simulink model "TRAMI_DCT_AT"  (R2018b)
settings: Solver=FixedStepDiscrete  StartTime=0.0  StopTime=88  FixedStep=10e-3  RelTol=1e-3  EnableMultiTasking=on
undefined symbols (not defined in the file): CONST_AP_GEAR_SUB_NEWTRAL, CONST_AP_IDLE_SPEED_CONT, CONST_AP_LOAD_SFT, CONST_AP_LOAD_SFT_HYS, CONST_CAR_WEIGHT, CONST_CL_NUM, CONST_F_DOWN_SYNCHRO, CONST_F_SYNCHRO, CONST_F_UP_SYNCHRO, CONST_FGR, CONST_I_FlYWHEEL, CONST_INATIA_CLANK, CONST_R_SHIFT_END_CD, CONST_R_SHIFT_END_EG, CONST_R_SHIFT_END_TD, CONST_R_SHIFT_END_UP, CONST_R_SYNCHRO_ENGAGE, CONST_R_TIRE, CONST_RATIO_TQ_REDUCTION, CONST_SKIP_SHIFT_MAX, CONST_SYN_NUM, CONST_T_SFT_END_EN, CONST_T_SFT_END_JUDGE, CONST_T_SFT_END_MAX, CONST_T_SFT_END_MIN, CONST_T_SHIFT_WAIT, CONST_T_TQ_PHASE_CD, CONST_T_TQ_PHASE_ND, CONST_T_TQ_PHASE_NR, CONST_T_TQ_PHASE_TD, CONST_T_TQ_PHASE_UP, CONST_TQ_CREEP_CONT, CONST_TQ_ENGAGE_CL_MARGIN, CONST_TQ_ENGAGE_CL_MIN, CONST_TQ_INATIA_TD_SHIFT, CONST_TQ_LOAD_SFT, CONST_TQ_LOAD_SFT_HYS, CONST_TQ_ND_ENGAGE, CONST_TQ_NR_ENGAGE, CONST_TQ_TQPHASE_MIN, CONST_V_IDLE_SPEED_CONT, Eng, FALSE, GrNP, GrRev, LoopTime, MAT_CL_ENGAGE, MAT_CL_SHARE_RATE, MAT_I_ACTUATOR, MAT_SYNCHRO_COM, MAT_T_GEAR_SUB_NEWTRAL, MAT_TRANS_MGR, MaxCL, Nm, PI, Shift_CD, Shift_ND, Shift_NR, Shift_TD, Shift_Up ... (+168)
libraries: simulink x26
(part 5 of 6)

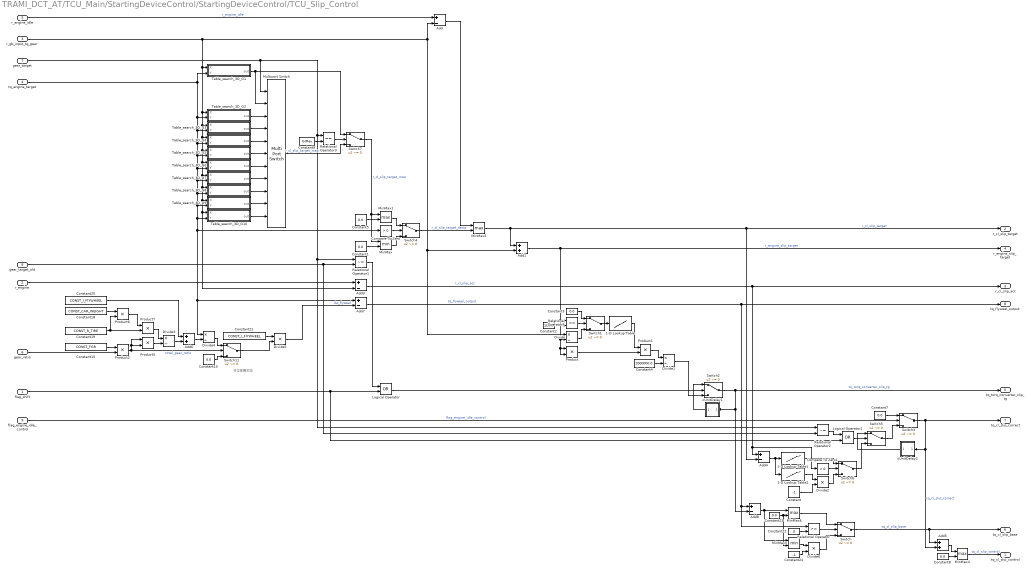
== system TRAMI_DCT_AT/TCU_Main/StartingDeviceControl/StartingDeviceControl/TCU_Slip_Control ==
  note: ゼロ除算対応
  flag_shift : Inport  OutDataTypeStr=boolean
      settings: AttributesFormatString=シフトフラグ[-]
  r_engine : Inport  Port=2  OutDataTypeStr=single
      settings: AttributesFormatString=エンジン回転数[rpm]
  r_gb_input_tg_gear : Inport  Port=3  OutDataTypeStr=single
      settings: AttributesFormatString=|
      | 目標ギヤ段でのGearBox入力回転
      | (GearBox出力回転から演算)[rpm]
  tq_engine_target : Inport  Port=4  OutDataTypeStr=single
      settings: AttributesFormatString=目標エンジントルク[Nm]
  r_engine_idle : Inport  Port=5  OutDataTypeStr=single
      settings: AttributesFormatString=エンジンアイドル回転数[rpm]
  gear_ratio : Inport  Port=6  OutDataTypeStr=single
      settings: AttributesFormatString=ギヤ比[-]
  gear_target : Inport  Port=7  OutDataTypeStr=int16
      settings: AttributesFormatString=目標ギヤ段[-]
  gear_target_old : Inport  Port=8  OutDataTypeStr=int16
      settings: AttributesFormatString=前回目標ギヤ段[-]
  flag_engine_idle_control : Inport  Port=9  OutDataTypeStr=boolean
      settings: AttributesFormatString=|
      | アイドル回転制御の実行判定フラグ
      | TRUE ：Engによるアイドル回転制御を実行
      | FALSE：クラッチスリップ制御によるEng回転制御を行う
      | [-]
  1-D Lookup Table : Lookup_n-D  NumberOfTableDimensions=1  BreakpointsForDimension1=T2D_COUPLING_CAP_FACT_X  Table=T2D_COUPLING_CAP_FACT_Y  InternalRulePriority=Speed  OutDataTypeStr=single  RndMeth=Simplest  InputSameDT=on
  1-D Lookup Table1 : Lookup_n-D  NumberOfTableDimensions=1  BreakpointsForDimension1=T2D_TQ_CL_SLIP_GAIN_X  Table=T2D_TQ_CL_SLIP_GAIN_Y  ExtrapMethod=Clip  InternalRulePriority=Speed  OutDataTypeStr=single  RndMeth=Simplest  InputSameDT=on
  1-D Lookup Table2 : Lookup_n-D  NumberOfTableDimensions=1  BreakpointsForDimension1=T2D_TQ_CL_SLIP_GAIN_X  Table=T2D_TQ_CL_SLIP_GAIN_Y  ExtrapMethod=Clip  InternalRulePriority=Speed  OutDataTypeStr=single  RndMeth=Simplest  InputSameDT=on
  Add{,3..4,8} (4 alike) : Sum  Inputs=+-  OutDataTypeStr=single
  Add1 : Sum  OutDataTypeStr=single
  Add5 : Sum  OutDataTypeStr=single
  Add6 : Sum  AccumDataTypeStr=single  OutDataTypeStr=single
  Add7 : Sum  Inputs=+-  AccumDataTypeStr=single  OutDataTypeStr=single
  Compare To Zero : simulink/Logic and Bit Operations/Compare To Zero  relop=>  OutDataTypeStr=boolean
  Compare To Zero1 : simulink/Logic and Bit Operations/Compare To Zero  relop=>  OutDataTypeStr=boolean
  Constant : Constant  Value=-1  OutDataTypeStr=single
  Constant{1,3,5,7..8,10,23} (7 alike) : Constant  Value=0.0  OutDataTypeStr=single
  Constant15 : Constant  Value=CONST_FGR  OutDataTypeStr=single
  Constant18 : Constant  Value=CONST_CAR_WEIGHT  OutDataTypeStr=single
  Constant19 : Constant  Value=CONST_R_TIRE  OutDataTypeStr=single
  Constant2 : Constant  Value=100.0  OutDataTypeStr=single
  Constant20 : Constant  Value=CONST_I_FlYWHEEL  OutDataTypeStr=single
  Constant21 : Constant  Value=CONST_I_FlYWHEEL  OutDataTypeStr=single
  Constant22 : Constant  Value=0  OutDataTypeStr=single
  Constant24 : Constant  Value=-1  OutDataTypeStr=single
  Constant4 : Constant  Value=1000000.0  OutDataTypeStr=single
  Constant9 : Constant  Value=GrRev  OutDataTypeStr=single
  Divide{,1,3..4} (4 alike) : Product  Inputs=*/  OutDataTypeStr=single
  Divide2 : Product  Inputs=**  OutDataTypeStr=single
  Divide5 : Product  Inputs=**  OutDataTypeStr=single
  Divide6 : Product  Inputs=**  OutDataTypeStr=single
  Logical Operator : Logic  Operator=OR  AllPortsSameDT=off  OutDataTypeStr=boolean
  Logical Operator1 : Logic  Operator=OR  AllPortsSameDT=off  OutDataTypeStr=boolean
  MinMax : MinMax  Inputs=2  OutDataTypeStr=single
  MinMax{1..2,4,6} (4 alike) : MinMax  Function=max  Inputs=2  OutDataTypeStr=single
  MinMax5 : MinMax  Inputs=2  OutDataTypeStr=single
  Multiport Switch : MultiPortSwitch  Inputs=9  DataPortForDefault=Additional data port  DiagnosticForDefault=None  OutDataTypeStr=single
  Product{,1..2,5..7} (6 alike) : Product  OutDataTypeStr=single
  Relational Operator : RelationalOperator  OutDataTypeStr=boolean  RndMeth=Simplest
  Relational Operator1 : RelationalOperator  Operator=~=  OutDataTypeStr=boolean  RndMeth=Nearest
  Relational Operator2 : RelationalOperator  Operator=~=  OutDataTypeStr=boolean  RndMeth=Nearest
  Relational Operator3 : RelationalOperator  Operator===  OutDataTypeStr=boolean  RndMeth=Simplest
  Relational Operator5 : RelationalOperator  Operator=<=  OutDataTypeStr=boolean  RndMeth=Nearest
  Switch{,1..7,11} (9 alike) : Switch  Criteria=u2 ~= 0  OutDataTypeStr=single
  Table_search_3D_G1 : Subsystem  mask(Table_search_3D){map=T3D_R_SLIP_G1, tbl_x=T2DX_R_SLIP_G1_Y, axis_x=T2DX_R_SLIP_G1_X, tbl_y=T2DY_R_SLIP_G1_Y, axis_y=T2DY_R_SLIP_G1_X}
      mask Display:
      | disp('Table_search_3D');
      | 
      | port_label('input',  1, 'X' );
      | port_label('input',  2, 'Y' );
      | port_label('output', 1, 'out' );
  Table_search_3D_G10 : Subsystem  mask(Table_search_3D){map=T3D_R_SLIP_G10, tbl_x=T2DX_R_SLIP_G10_Y, axis_x=T2DX_R_SLIP_G10_X, tbl_y=T2DY_R_SLIP_G10_Y, axis_y=T2DY_R_SLIP_G10_X}
      mask Display:
      | disp('Table_search_3D');
      | 
      | port_label('input',  1, 'X' );
      | port_label('input',  2, 'Y' );
      | port_label('output', 1, 'out' );
  Table_search_3D_G2 : Subsystem  mask(Table_search_3D){map=T3D_R_SLIP_G2, tbl_x=T2DX_R_SLIP_G2_Y, axis_x=T2DX_R_SLIP_G2_X, tbl_y=T2DY_R_SLIP_G2_Y, axis_y=T2DY_R_SLIP_G2_X}
      mask Display:
      | disp('Table_search_3D');
      | 
      | port_label('input',  1, 'X' );
      | port_label('input',  2, 'Y' );
      | port_label('output', 1, 'out' );
  Table_search_3D_G3 : Subsystem  mask(Table_search_3D){map=T3D_R_SLIP_G3, tbl_x=T2DX_R_SLIP_G3_Y, axis_x=T2DX_R_SLIP_G3_X, tbl_y=T2DY_R_SLIP_G3_Y, axis_y=T2DY_R_SLIP_G3_X}
      mask Display:
      | disp('Table_search_3D');
      | 
      | port_label('input',  1, 'X' );
      | port_label('input',  2, 'Y' );
      | port_label('output', 1, 'out' );
  Table_search_3D_G4 : Subsystem  mask(Table_search_3D){map=T3D_R_SLIP_G4, tbl_x=T2DX_R_SLIP_G4_Y, axis_x=T2DX_R_SLIP_G4_X, tbl_y=T2DY_R_SLIP_G4_Y, axis_y=T2DY_R_SLIP_G4_X}
      mask Display:
      | disp('Table_search_3D');
      | 
      | port_label('input',  1, 'X' );
      | port_label('input',  2, 'Y' );
      | port_label('output', 1, 'out' );
  Table_search_3D_G5 : Subsystem  mask(Table_search_3D){map=T3D_R_SLIP_G5, tbl_x=T2DX_R_SLIP_G5_Y, axis_x=T2DX_R_SLIP_G5_X, tbl_y=T2DY_R_SLIP_G5_Y, axis_y=T2DY_R_SLIP_G5_X}
      mask Display:
      | disp('Table_search_3D');
      | 
      | port_label('input',  1, 'X' );
      | port_label('input',  2, 'Y' );
      | port_label('output', 1, 'out' );
  Table_search_3D_G6 : Subsystem  mask(Table_search_3D){map=T3D_R_SLIP_G6, tbl_x=T2DX_R_SLIP_G6_Y, axis_x=T2DX_R_SLIP_G6_X, tbl_y=T2DY_R_SLIP_G6_Y, axis_y=T2DY_R_SLIP_G6_X}
      mask Display:
      | disp('Table_search_3D');
      | 
      | port_label('input',  1, 'X' );
      | port_label('input',  2, 'Y' );
      | port_label('output', 1, 'out' );
  Table_search_3D_G7 : Subsystem  mask(Table_search_3D){map=T3D_R_SLIP_G7, tbl_x=T2DX_R_SLIP_G7_Y, axis_x=T2DX_R_SLIP_G7_X, tbl_y=T2DY_R_SLIP_G7_Y, axis_y=T2DY_R_SLIP_G7_X}
      mask Display:
      | disp('Table_search_3D');
      | 
      | port_label('input',  1, 'X' );
      | port_label('input',  2, 'Y' );
      | port_label('output', 1, 'out' );
  Table_search_3D_G8 : Subsystem  mask(Table_search_3D){map=T3D_R_SLIP_G8, tbl_x=T2DX_R_SLIP_G8_Y, axis_x=T2DX_R_SLIP_G8_X, tbl_y=T2DY_R_SLIP_G8_Y, axis_y=T2DY_R_SLIP_G8_X}
      mask Display:
      | disp('Table_search_3D');
      | 
      | port_label('input',  1, 'X' );
      | port_label('input',  2, 'Y' );
      | port_label('output', 1, 'out' );
  Table_search_3D_G9 : Subsystem  mask(Table_search_3D){map=T3D_R_SLIP_G9, tbl_x=T2DX_R_SLIP_G9_Y, axis_x=T2DX_R_SLIP_G9_X, tbl_y=T2DY_R_SLIP_G9_Y, axis_y=T2DY_R_SLIP_G9_X}
      mask Display:
      | disp('Table_search_3D');
      | 
      | port_label('input',  1, 'X' );
      | port_label('input',  2, 'Y' );
      | port_label('output', 1, 'out' );
  cUnitDelay1 : Subsystem  mask(resetable_unit_delay){initParam=0}
      mask prompts: initParam "初期化値"
      mask Display: dpoly(1,[1,0],'z')
  cUnitDelay2 : Subsystem  mask(resetable_unit_delay){initParam=0}
      mask prompts: initParam "初期化値"
      mask Display: dpoly(1,[1,0],'z')
  tq_cl_slip_control : Outport  OutDataTypeStr=single
      settings: AttributesFormatString=スリップ制御クラッチのトルク容量[Nm]
  r_cl_slip_target : Outport  Port=2  OutDataTypeStr=single
      settings: AttributesFormatString=目標スリップ量[rpm]
  r_cl_slip_act : Outport  Port=3  OutDataTypeStr=single
      settings: AttributesFormatString=実スリップ量[rpm]
  r_engine_slip_target : Outport  Port=4  OutDataTypeStr=single
      settings: AttributesFormatString=目標エンジン回転[rpm]
  tq_torq_converter_slip_tg : Outport  Port=5  OutDataTypeStr=single
      settings: AttributesFormatString=目標スリップ時の流体伝達トルク[Nm]
  tq_cl_slip_base : Outport  Port=6  OutDataTypeStr=single
      settings: AttributesFormatString=スリップクラッチのトルク容量基準値[Nm]
  tq_cl_slip_correct : Outport  Port=7  OutDataTypeStr=single
      settings: AttributesFormatString=クラッチトルクの補正値[Nm]
  tq_flyweel_output : Outport  Port=8  OutDataTypeStr=single
      settings: AttributesFormatString=イナーシャを考慮したフライホイール出力トルク[Nm]
  wires:
  r_gb_input_tg_gear/1 -> Add3/2, Table_search_3D_G10/1(X), Table_search_3D_G9/1(X), Table_search_3D_G8/1(X), Table_search_3D_G7/1(X), Table_search_3D_G6/1(X), Table_search_3D_G5/1(X), Table_search_3D_G4/1(X), Table_search_3D_G3/1(X), Table_search_3D_G2/1(X), Table_search_3D_G1/1(X), Add1/2, Divide/1, Add/2
  gear_target/1 -> Multiport Switch/1, Relational Operator1/1, Relational Operator2/1, Relational Operator3/1
  Table_search_3D_G1/1(out) -> Multiport Switch/2, Switch7/1
  Table_search_3D_G2/1(out) -> Multiport Switch/3
  Table_search_3D_G3/1(out) -> Multiport Switch/4
  Table_search_3D_G4/1(out) -> Multiport Switch/5
  Table_search_3D_G5/1(out) -> Multiport Switch/6
  Table_search_3D_G6/1(out) -> Multiport Switch/7
  Table_search_3D_G7/1(out) -> Multiport Switch/8
  Table_search_3D_G8/1(out) -> Multiport Switch/9
  Table_search_3D_G9/1(out) -> Multiport Switch/10
  Table_search_3D_G10/1(out) -> Multiport Switch/11
  tq_engine_target/1 -> Compare To Zero/1, Divide4/1, Add7/1, Table_search_3D_G10/2(Y), Table_search_3D_G9/2(Y), Table_search_3D_G8/2(Y), Table_search_3D_G7/2(Y), Table_search_3D_G6/2(Y), Table_search_3D_G5/2(Y), Table_search_3D_G4/2(Y), Table_search_3D_G3/2(Y), Table_search_3D_G2/2(Y), Table_search_3D_G1/2(Y)
  Switch7/1 -> MinMax/1, MinMax1/1  "r_cl_slip_target_map"
  Compare To Zero/1 -> Switch4/2
  MinMax1/1 -> Switch4/1
  MinMax/1 -> Switch4/3
  Constant5/1 -> MinMax1/2
  Constant1/1 -> MinMax/2
  Switch4/1 -> MinMax2/2  "r_cl_slip_target_temp"
  Add/1 -> MinMax2/1
  r_engine_idle/1 -> Add/1  "r_engine_idle"
  Add1/1 -> r_engine_slip_target/1, Relational Operator5/1, Product/2, Product/1, Divide/2  "r_engine_slip_target"
  Constant2/1 -> Relational Operator5/2
  Relational Operator5/1 -> Switch1/2
  Constant3/1 -> Switch1/1
  Switch1/1 -> 1-D Lookup Table/1
  Divide/1 -> Switch1/3
  1-D Lookup Table/1 -> Product1/1
  Relational Operator1/1 -> Logical Operator/1
  flag_shift/1 -> Logical Operator/2, Logical Operator1/2
  Logical Operator/1 -> Switch2/2
  Switch2/1 -> cUnitDelay1/1(<param>), Add8/2, tq_torq_converter_slip_tg/1  "tq_torq_converter_slip_tg"
  Product1/1 -> Divide1/1
  Constant4/1 -> Divide1/2
  Product/1 -> Product1/2
  Divide1/1 -> Switch2/3
  r_engine/1 -> Add3/1
  Switch3/1 -> tq_cl_slip_correct/1, Add5/2, cUnitDelay2/1(<param>)  "tq_cl_slip_correct"
  Switch5/1 -> Switch3/3
  Switch6/1 -> Switch5/3
  flag_engine_idle_control/1 -> Switch3/2  "flag_engine_idle_control"
  Constant7/1 -> Switch3/1
  cUnitDelay2/1(preParam) -> Switch5/1
  Logical Operator1/1 -> Switch5/2
  Relational Operator2/1 -> Logical Operator1/1
  Compare To Zero1/1 -> Switch6/2
  Add3/1 -> r_cl_slip_act/1, Compare To Zero1/1, Add4/1  "r_cl_slip_act"
  1-D Lookup Table2/1 -> Divide2/1
  Add4/1 -> 1-D Lookup Table1/1, 1-D Lookup Table2/1
  MinMax2/1 -> r_cl_slip_target/1, Add4/2, Add1/1  "r_cl_slip_target"
  MinMax4/1 -> tq_cl_slip_control/1  "tq_cl_slip_control"
  Add5/1 -> MinMax4/1
  Constant8/1 -> MinMax4/2
  gear_target_old/1 -> Relational Operator2/2, Relational Operator1/2
  Constant/1 -> Divide2/2
  Divide2/1 -> Switch6/3
  1-D Lookup Table1/1 -> Switch6/1
  Constant15/1 -> Product2/1
  gear_ratio/1 -> Product2/2
  Add6/1 -> Divide4/2
  Product2/1 -> Product5/1, Product5/2, Switch11/2  "total_gear_ratio"
  Constant18/1 -> Product6/1
  Constant19/1 -> Product6/2, Product7/2
  Product6/1 -> Product7/1
  Product7/1 -> Divide3/1
  Constant20/1 -> Add6/1
  Switch11/1 -> Divide5/2
  Constant21/1 -> Divide5/1
  Divide5/1 -> Add7/2  "dw_flyweel"
  Add7/1 -> tq_flyweel_output/1, Add8/1, Relational Operator/1  "tq_flyweel_output"
  Relational Operator/1 -> Switch/2
  Constant22/1 -> Relational Operator/2
  MinMax6/1 -> Switch/1
  Divide6/1 -> Switch/3
  Add8/1 -> MinMax6/1, MinMax5/1
  Constant23/1 -> MinMax5/2, MinMax6/2
  Constant24/1 -> Divide6/2
  MinMax5/1 -> Divide6/1
  Switch/1 -> tq_cl_slip_base/1, Add5/1  "tq_cl_slip_base"
  Divide3/1 -> Add6/2
  Product5/1 -> Divide3/2
  Divide4/1 -> Switch11/1
  cUnitDelay1/1(preParam) -> Switch2/1
  Relational Operator3/1 -> Switch7/2
  Constant9/1 -> Relational Operator3/2
  Multiport Switch/1 -> Switch7/3  "r_cl_slip_target_map"
  Constant10/1 -> Switch11/3

== system TRAMI_DCT_AT/TCU_Main/StartingDeviceControl/StartingDeviceControl/TCU_Torque_Input_GearBox ==
  tq_engine_target : Inport  OutDataTypeStr=single
      settings: AttributesFormatString=目標エンジントルク[Nm]
  torq_ratio_torq_converter : Inport  Port=2  OutDataTypeStr=single
      settings: AttributesFormatString=トルク比[-]
  Divide : Product  Inputs=**  OutDataTypeStr=single
  tq_gearbox_input : Outport  OutDataTypeStr=single
      settings: AttributesFormatString=ギヤボックス入力トルク[Nm]
  wires:
  tq_engine_target/1 -> Divide/1
  torq_ratio_torq_converter/1 -> Divide/2
  Divide/1 -> tq_gearbox_input/1  "tq_gearbox_input"

== system TRAMI_DCT_AT/TCU_Main/AccControl/AccControl/TCU_EOP_Control/Table_search_3D_sample6 ==
  X : Inport  OutDataTypeStr=single
  Y : Inport  Port=2  OutDataTypeStr=single
  1-D Lookup Table1 : Lookup_n-D  NumberOfTableDimensions=1  BreakpointsForDimension1=axis_x  Table=tbl_x  ExtrapMethod=Clip  InternalRulePriority=Speed  OutDataTypeStr=single  RndMeth=Simplest  InputSameDT=on
  1-D Lookup Table2 : Lookup_n-D  NumberOfTableDimensions=1  BreakpointsForDimension1=axis_y  Table=tbl_y  ExtrapMethod=Clip  InternalRulePriority=Speed  OutDataTypeStr=single  RndMeth=Simplest  InputSameDT=on
  2-D Lookup Table : Lookup_n-D  BreakpointsForDimension1=tbl_y  BreakpointsForDimension2=tbl_x  Table=map  ExtrapMethod=Clip  InternalRulePriority=Speed  OutDataTypeStr=single  RndMeth=Simplest  InputSameDT=on
  out : Outport  OutDataTypeStr=single
  wires:
  1-D Lookup Table1/1 -> 2-D Lookup Table/2  "x_nrm"
  1-D Lookup Table2/1 -> 2-D Lookup Table/1  "y_nrm"
  Y/1 -> 1-D Lookup Table2/1  "data_y"
  X/1 -> 1-D Lookup Table1/1  "data_x"
  2-D Lookup Table/1 -> out/1

== system TRAMI_DCT_AT/TCU_Main/ClutchControl/ClutchControl/TCU_Gear_Clutch_Control/cUnitDelay2 ==
  <param> : Inport
  Constant13 : Constant  Value=initParam  OutDataTypeStr=int16
  Switch12 : Switch  Criteria=u2 > Threshold
  Unit Delay2 : UnitDelay  InitialCondition=zeros(size(initParam))  SampleTime=-1
  preParam : Outport
  wires:
  Unit Delay2/1 -> Switch12/3
  Switch12/1 -> preParam/1
  [FlagInit] -> Switch12/2
  Constant13/1 -> Switch12/1
  <param>/1 -> Unit Delay2/1

== system TRAMI_DCT_AT/TCU_Main/ClutchControl/ClutchControl/TCU_SYNCHORO_CONTROL_AT_DCT/TCU_SYNCHORO_CONTROL_AT ==
  gear_target : Inport  OutDataTypeStr=int16
      settings: AttributesFormatString=目標ギヤ段[-]
  gear_before_shift : Inport  Port=2  OutDataTypeStr=int16
      settings: AttributesFormatString=変速前ギヤ段[-]
  gear_sub1 : Inport  Port=3  OutDataTypeStr=int16
      settings: AttributesFormatString=待機ギヤ段（奇数軸）[-]
  gear_sub2 : Inport  Port=4  OutDataTypeStr=int16
      settings: AttributesFormatString=待機ギヤ段（偶数軸）[-]
  f_synchro_old : Inport  Port=5  OutDataTypeStr=single
      settings: AttributesFormatString=前回のシンクロの押し力[N]
  Constant1 : Constant  Value=[0 0 0 0 0 0 0 0 0 0]  OutDataTypeStr=single
  Constant13 : Constant  Value=FALSE  OutDataTypeStr=boolean
  Terminator{,1..4} (5 alike) : Terminator
  f_synchro : Outport  OutDataTypeStr=single
      settings: AttributesFormatString=シンクロの押し力[N]
  flag_synchro_com : Outport  Port=2  OutDataTypeStr=boolean
      settings: AttributesFormatString=シンクロ締結指示[-]
  wires:
  gear_before_shift/1 -> Terminator1/1
  gear_target/1 -> Terminator/1
  Constant13/1 -> flag_synchro_com/1  "flag_synchro_com"
  Constant1/1 -> f_synchro/1  "f_synchro"
  gear_sub1/1 -> Terminator2/1
  gear_sub2/1 -> Terminator3/1
  f_synchro_old/1 -> Terminator4/1

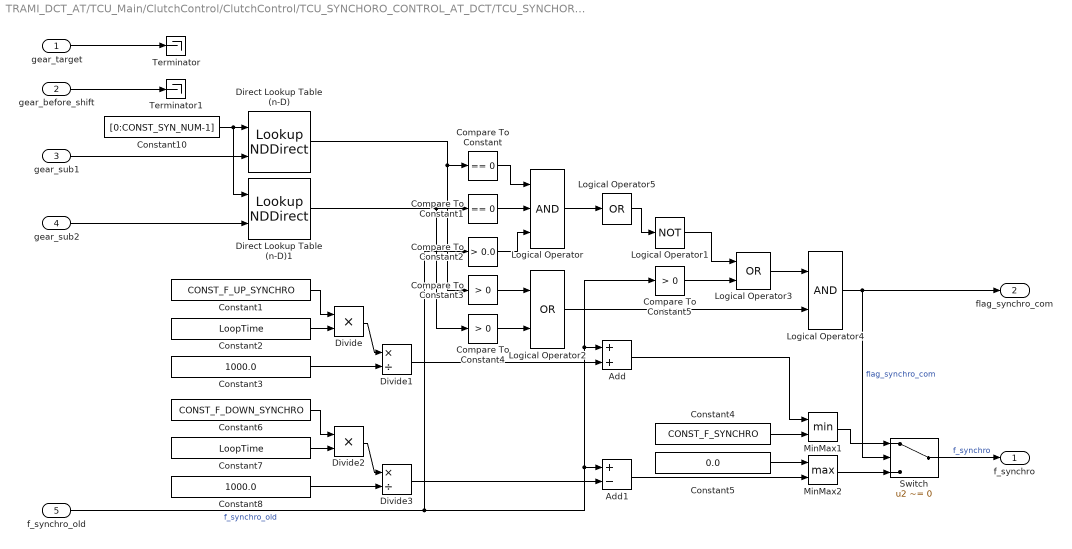
== system TRAMI_DCT_AT/TCU_Main/ClutchControl/ClutchControl/TCU_SYNCHORO_CONTROL_AT_DCT/TCU_SYNCHORO_CONTROL_DCT ==
  gear_target : Inport  OutDataTypeStr=int16
      settings: AttributesFormatString=目標ギヤ段[-]
  gear_before_shift : Inport  Port=2  OutDataTypeStr=int16
      settings: AttributesFormatString=変速前ギヤ段[-]
  gear_sub1 : Inport  Port=3  OutDataTypeStr=int16
      settings: AttributesFormatString=待機ギヤ段（奇数軸）[-]
  gear_sub2 : Inport  Port=4  OutDataTypeStr=int16
      settings: AttributesFormatString=待機ギヤ段（偶数軸）[-]
  f_synchro_old : Inport  Port=5  OutDataTypeStr=single
      settings: AttributesFormatString=前回のシンクロの押し力[N]
  Add : Sum  OutDataTypeStr=single
  Add1 : Sum  Inputs=+-  OutDataTypeStr=single
  Compare To Constant : simulink/Logic and Bit Operations/Compare To Constant  relop===  const=0  OutDataTypeStr=boolean
  Compare To Constant1 : simulink/Logic and Bit Operations/Compare To Constant  relop===  const=0  OutDataTypeStr=boolean
  Compare To Constant2 : simulink/Logic and Bit Operations/Compare To Constant  relop=>  const=0.0  OutDataTypeStr=boolean
  Compare To Constant3 : simulink/Logic and Bit Operations/Compare To Constant  relop=>  const=0  OutDataTypeStr=boolean
  Compare To Constant4 : simulink/Logic and Bit Operations/Compare To Constant  relop=>  const=0  OutDataTypeStr=boolean
  Compare To Constant5 : simulink/Logic and Bit Operations/Compare To Constant  relop=>  const=0  OutDataTypeStr=boolean
  Constant1 : Constant  Value=CONST_F_UP_SYNCHRO  OutDataTypeStr=single
  Constant10 : Constant  Value=[0:CONST_SYN_NUM-1]  OutDataTypeStr=int16
  Constant2 : Constant  Value=LoopTime  OutDataTypeStr=single
  Constant3 : Constant  Value=1000.0  OutDataTypeStr=single
  Constant4 : Constant  Value=CONST_F_SYNCHRO  OutDataTypeStr=single
  Constant5 : Constant  Value=0.0  OutDataTypeStr=single
  Constant6 : Constant  Value=CONST_F_DOWN_SYNCHRO  OutDataTypeStr=single
  Constant7 : Constant  Value=LoopTime  OutDataTypeStr=single
  Constant8 : Constant  Value=1000.0  OutDataTypeStr=single
  Direct Lookup Table (n-D) : LookupNDDirect  Table=MAT_SYNCHRO_COM
  Direct Lookup Table (n-D)1 : LookupNDDirect  Table=MAT_SYNCHRO_COM
  Divide : Product  OutDataTypeStr=single
  Divide1 : Product  Inputs=*/  OutDataTypeStr=single
  Divide2 : Product  OutDataTypeStr=single
  Divide3 : Product  Inputs=*/  OutDataTypeStr=single
  Logical Operator : Logic  Inputs=3  AllPortsSameDT=off  OutDataTypeStr=boolean
  Logical Operator1 : Logic  Operator=NOT  Inputs=3  AllPortsSameDT=off  OutDataTypeStr=boolean
  Logical Operator2 : Logic  Operator=OR  AllPortsSameDT=off  OutDataTypeStr=boolean
  Logical Operator3 : Logic  Operator=OR  AllPortsSameDT=off  OutDataTypeStr=boolean
  Logical Operator4 : Logic  AllPortsSameDT=off  OutDataTypeStr=boolean
  Logical Operator5 : Logic  Operator=OR  Inputs=1  AllPortsSameDT=off  OutDataTypeStr=boolean
  MinMax1 : MinMax  Inputs=2  OutDataTypeStr=single
  MinMax2 : MinMax  Function=max  Inputs=2  OutDataTypeStr=single
  Switch : Switch  Criteria=u2 ~= 0  OutDataTypeStr=single  ZeroCross=off
  Terminator : Terminator
  Terminator1 : Terminator
  f_synchro : Outport  OutDataTypeStr=single
      settings: AttributesFormatString=シンクロの押し力[N]
  flag_synchro_com : Outport  Port=2  OutDataTypeStr=boolean
      settings: AttributesFormatString=シンクロ締結指示[-]
  wires:
  Constant5/1 -> MinMax2/1
  Logical Operator4/1 -> Switch/2, flag_synchro_com/1  "flag_synchro_com"
  Constant3/1 -> Divide1/2
  Compare To Constant4/1 -> Logical Operator2/2
  Constant8/1 -> Divide3/2
  Logical Operator1/1 -> Logical Operator3/1
  Logical Operator5/1 -> Logical Operator1/1
  gear_target/1 -> Terminator/1
  Compare To Constant2/1 -> Logical Operator/3
  gear_before_shift/1 -> Terminator1/1
  Compare To Constant1/1 -> Logical Operator/2
  Compare To Constant3/1 -> Logical Operator2/1
  Switch/1 -> f_synchro/1  "f_synchro"
  Direct Lookup Table (n-D)/1 -> Compare To Constant3/1, Compare To Constant/1
  Logical Operator2/1 -> Logical Operator4/2
  Constant1/1 -> Divide/1
  Divide2/1 -> Divide3/1
  Constant10/1 -> Direct Lookup Table (n-D)/1, Direct Lookup Table (n-D)1/1
  Constant6/1 -> Divide2/1
  gear_sub2/1 -> Direct Lookup Table (n-D)1/2
  gear_sub1/1 -> Direct Lookup Table (n-D)/2
  Constant7/1 -> Divide2/2
  Add/1 -> MinMax1/1
  Compare To Constant/1 -> Logical Operator/1
  Add1/1 -> MinMax2/2
  Logical Operator3/1 -> Logical Operator4/1
  Compare To Constant5/1 -> Logical Operator3/2
  Divide3/1 -> Add1/2
  Direct Lookup Table (n-D)1/1 -> Compare To Constant4/1, Compare To Constant1/1
  Divide1/1 -> Add/2
  Constant4/1 -> MinMax1/2
  MinMax2/1 -> Switch/3
  MinMax1/1 -> Switch/1
  Logical Operator/1 -> Logical Operator5/1
  Divide/1 -> Divide1/1
  f_synchro_old/1 -> Compare To Constant5/1, Add/1, Add1/1, Compare To Constant2/1  "f_synchro_old"
  Constant2/1 -> Divide/2

== system TRAMI_DCT_AT/TCU_Main/ClutchControl/ClutchControl/TCU_SYNCHORO_STATUS_AT_DCT/TCU_SYNCHORO_STATUS_AT ==
  gear_target : Inport  OutDataTypeStr=int16
      settings: AttributesFormatString=目標ギヤ段[-]
  f_synchro : Inport  Port=2  OutDataTypeStr=single
      settings: AttributesFormatString=シンクロの押し力[N]
  r_synchoro_dif : Inport  Port=3  OutDataTypeStr=single
      settings: AttributesFormatString=各シンクロ差回転[rpm]
  Constant : Constant  Value=TRUE  OutDataTypeStr=boolean
  Terminator : Terminator
  Terminator1 : Terminator
  Terminator2 : Terminator
  flag_synchro_ready : Outport  OutDataTypeStr=boolean
      settings: AttributesFormatString=全シンクロの同期判定[-]
  wires:
  Constant/1 -> flag_synchro_ready/1  "flag_synchro_ready"
  gear_target/1 -> Terminator/1  "gear_target"
  f_synchro/1 -> Terminator1/1  "f_synchro"
  r_synchoro_dif/1 -> Terminator2/1  "r_synchoro_dif"

== system TRAMI_DCT_AT/TCU_Main/ClutchControl/ClutchControl/TCU_SYNCHORO_STATUS_AT_DCT/TCU_SYNCHORO_STATUS_DCT ==
  gear_target : Inport  OutDataTypeStr=int16
      settings: AttributesFormatString=目標ギヤ段[-]
  f_synchro : Inport  Port=2  OutDataTypeStr=single
      settings: AttributesFormatString=シンクロの押し力[N]
  r_synchoro_dif : Inport  Port=3  OutDataTypeStr=single
      settings: AttributesFormatString=各シンクロ差回転[rpm]
  Abs : Abs  OutDataTypeStr=single
  Compare To Constant : simulink/Logic and Bit Operations/Compare To Constant  relop=>  const=0  OutDataTypeStr=boolean
  Constant10 : Constant  Value=CONST_R_SYNCHRO_ENGAGE  OutDataTypeStr=single
  Constant3 : Constant  Value=[0:CONST_SYN_NUM-1]  OutDataTypeStr=int16
  Constant9 : Constant  Value=CONST_F_SYNCHRO  OutDataTypeStr=single
  Direct Lookup Table (n-D) : LookupNDDirect  Table=MAT_SYNCHRO_COM
  Logical Operator : Logic  AllPortsSameDT=off  OutDataTypeStr=boolean
  Logical Operator1 : Logic  Operator=NOT  Inputs=3  AllPortsSameDT=off  OutDataTypeStr=boolean
  Logical Operator5 : Logic  Operator=OR  Inputs=1  AllPortsSameDT=off  OutDataTypeStr=boolean
  Logical Operator6 : Logic  Operator=OR  AllPortsSameDT=off  OutDataTypeStr=boolean
  Relational Operator : RelationalOperator  Operator=<  OutDataTypeStr=boolean  RndMeth=Nearest
  Relational Operator1 : RelationalOperator  Operator=>  OutDataTypeStr=boolean  RndMeth=Nearest
  Selector1 : Selector  InputPortWidth=MaxSyn  IndexOptions=Index vector (dialog)  Indices=[1:CONST_SYN_NUM]  OutputSizes=1
  flag_synchro_ready : Outport  OutDataTypeStr=boolean
      settings: AttributesFormatString=全シンクロの同期判定[-]
  wires:
  r_synchoro_dif/1 -> Selector1/1  "r_synchoro_dif"
  Logical Operator/1 -> Logical Operator5/1
  Logical Operator5/1 -> Logical Operator1/1
  Logical Operator6/1 -> Logical Operator/2
  Logical Operator1/1 -> flag_synchro_ready/1  "flag_synchro_ready"
  Constant3/1 -> Direct Lookup Table (n-D)/1
  gear_target/1 -> Direct Lookup Table (n-D)/2  "gear_target"
  Relational Operator1/1 -> Logical Operator6/2
  Constant10/1 -> Relational Operator1/2
  f_synchro/1 -> Relational Operator/1  "f_synchro"
  Relational Operator/1 -> Logical Operator6/1
  Compare To Constant/1 -> Logical Operator/1
  Abs/1 -> Relational Operator1/1
  Constant9/1 -> Relational Operator/2
  Direct Lookup Table (n-D)/1 -> Compare To Constant/1
  Selector1/1 -> Abs/1

== system TRAMI_DCT_AT/TCU_Main/ClutchControl/ClutchControl/TCU_Shift_Inertia_Torq/cUnitDelay1 ==
  <param> : Inport
  Constant13 : Constant  Value=initParam  OutDataTypeStr=single
  Switch12 : Switch  Criteria=u2 > Threshold
  Unit Delay2 : UnitDelay  InitialCondition=zeros(size(initParam))  SampleTime=-1
  preParam : Outport
  wires:
  Unit Delay2/1 -> Switch12/3
  Switch12/1 -> preParam/1
  [FlagInit] -> Switch12/2
  Constant13/1 -> Switch12/1
  <param>/1 -> Unit Delay2/1

== system TRAMI_DCT_AT/TCU_Main/ClutchControl/ClutchControl/TCU_Shift_Inertia_Torq/cUnitDelay2 ==
  <param> : Inport
  Constant13 : Constant  Value=initParam  OutDataTypeStr=single
  Switch12 : Switch  Criteria=u2 > Threshold
  Unit Delay2 : UnitDelay  InitialCondition=zeros(size(initParam))  SampleTime=-1
  preParam : Outport
  wires:
  Unit Delay2/1 -> Switch12/3
  Switch12/1 -> preParam/1
  [FlagInit] -> Switch12/2
  Constant13/1 -> Switch12/1
  <param>/1 -> Unit Delay2/1

== system TRAMI_DCT_AT/TCU_Main/ClutchControl/ClutchControl/TCU_Shift_Inertia_Torq/cUnitDelay3 ==
  <param> : Inport
  Constant13 : Constant  Value=initParam  OutDataTypeStr=int16
  Switch12 : Switch  Criteria=u2 > Threshold
  Unit Delay2 : UnitDelay  InitialCondition=zeros(size(initParam))  SampleTime=-1
  preParam : Outport
  wires:
  <param>/1 -> Unit Delay2/1
  Constant13/1 -> Switch12/1
  [FlagInit] -> Switch12/2
  Switch12/1 -> preParam/1
  Unit Delay2/1 -> Switch12/3

== system TRAMI_DCT_AT/TCU_Main/ClutchControl/ClutchControl/TCU_Shift_Inertia_Torq/cUnitDelay4 ==
  <param> : Inport
  Constant13 : Constant  Value=initParam  OutDataTypeStr=single
  Switch12 : Switch  Criteria=u2 > Threshold
  Unit Delay2 : UnitDelay  InitialCondition=zeros(size(initParam))  SampleTime=-1
  preParam : Outport
  wires:
  <param>/1 -> Unit Delay2/1
  Constant13/1 -> Switch12/1
  [FlagInit] -> Switch12/2
  Switch12/1 -> preParam/1
  Unit Delay2/1 -> Switch12/3

== system TRAMI_DCT_AT/TCU_Main/GearControl/GearControl/TCU_Up_Shift_Torque_Reduction/cUnitDelay2 ==
  <param> : Inport
  Constant13 : Constant  Value=initParam  OutDataTypeStr=boolean
  Switch12 : Switch  Criteria=u2 > Threshold
  Unit Delay2 : UnitDelay  InitialCondition=zeros(size(initParam))  SampleTime=-1
  preParam : Outport
  wires:
  Unit Delay2/1 -> Switch12/3
  Switch12/1 -> preParam/1
  [FlagInit] -> Switch12/2
  Constant13/1 -> Switch12/1
  <param>/1 -> Unit Delay2/1

== system TRAMI_DCT_AT/TCU_Main/ShiftScheduleControl/ShiftScheduleControl/TCU_Gear_Shift_Type/cUnitDelay2 ==
  <param> : Inport
  Constant13 : Constant  Value=initParam  OutDataTypeStr=single
  Switch12 : Switch  Criteria=u2 > Threshold
  Unit Delay2 : UnitDelay  InitialCondition=zeros(size(initParam))  SampleTime=-1
  preParam : Outport
  wires:
  Unit Delay2/1 -> Switch12/3
  Switch12/1 -> preParam/1
  [FlagInit] -> Switch12/2
  Constant13/1 -> Switch12/1
  <param>/1 -> Unit Delay2/1

== system TRAMI_DCT_AT/TCU_Main/ShiftScheduleControl/ShiftScheduleControl/TCU_Gear_Target/cUnitDelay2 ==
  <param> : Inport
  Constant13 : Constant  Value=initParam  OutDataTypeStr=single
  Switch12 : Switch  Criteria=u2 > Threshold
  Unit Delay2 : UnitDelay  InitialCondition=zeros(size(initParam))  SampleTime=-1
  preParam : Outport
  wires:
  Unit Delay2/1 -> Switch12/3
  Switch12/1 -> preParam/1
  [FlagInit] -> Switch12/2
  Constant13/1 -> Switch12/1
  <param>/1 -> Unit Delay2/1

== system TRAMI_DCT_AT/TCU_Main/ShiftScheduleControl/ShiftScheduleControl/TCU_Gear_Target/calc_gear_target ==
  j : Inport  OutDataTypeStr=int16
  gear_before_shift : Inport  Port=2  OutDataTypeStr=int16
  Add : Sum  Inputs=+-  OutDataTypeStr=int16
  for_Outer_loop : Subsystem
  gear_target : Outport  OutDataTypeStr=int16
  wires:
  for_Outer_loop/1(gear_target) -> gear_target/1
  gear_before_shift/1 -> Add/1, for_Outer_loop/2(gear_before_shift)
  j/1 -> Add/2, for_Outer_loop/1(j)
  Add/1 -> for_Outer_loop/3(NUM_LOOP)

== system TRAMI_DCT_AT/TCU_Main/ShiftScheduleControl/ShiftScheduleControl/TCU_Load_shift/Switch_with_hys ==
  flag_old : Inport  OutDataTypeStr=boolean
  val : Inport  Port=2  OutDataTypeStr=single
  cal : Inport  Port=3  OutDataTypeStr=single
  hys : Inport  Port=4  OutDataTypeStr=single
  Add : Sum  Inputs=+-  OutDataTypeStr=single
  Constant : Constant  Value=TRUE  OutDataTypeStr=boolean
  Constant1 : Constant  Value=FALSE  OutDataTypeStr=boolean
  Relational Operator1 : RelationalOperator  Operator=<  OutDataTypeStr=boolean  RndMeth=Nearest
  Relational Operator3 : RelationalOperator  OutDataTypeStr=boolean  RndMeth=Nearest
  Switch1 : Switch  Criteria=u2 ~= 0  OutDataTypeStr=boolean
  Switch2 : Switch  Criteria=u2 ~= 0  OutDataTypeStr=boolean
  flag : Outport  OutDataTypeStr=boolean
  wires:
  val/1 -> Relational Operator1/1, Relational Operator3/1
  cal/1 -> Relational Operator3/2, Add/1
  Relational Operator3/1 -> Switch1/2
  Constant/1 -> Switch1/1
  Switch2/1 -> Switch1/3
  Relational Operator1/1 -> Switch2/2
  Add/1 -> Relational Operator1/2
  hys/1 -> Add/2
  Constant1/1 -> Switch2/1
  Switch1/1 -> flag/1
  flag_old/1 -> Switch2/3

== system TRAMI_DCT_AT/TCU_Main/ShiftScheduleControl/ShiftScheduleControl/TCU_Load_shift/Switch_with_hys1 ==
  flag_old : Inport  OutDataTypeStr=boolean
  val : Inport  Port=2  OutDataTypeStr=single
  cal : Inport  Port=3  OutDataTypeStr=single
  hys : Inport  Port=4  OutDataTypeStr=single
  Add : Sum  Inputs=+-  OutDataTypeStr=single
  Constant : Constant  Value=TRUE  OutDataTypeStr=boolean
  Constant1 : Constant  Value=FALSE  OutDataTypeStr=boolean
  Relational Operator1 : RelationalOperator  Operator=<  OutDataTypeStr=boolean  RndMeth=Nearest
  Relational Operator3 : RelationalOperator  OutDataTypeStr=boolean  RndMeth=Nearest
  Switch1 : Switch  Criteria=u2 ~= 0  OutDataTypeStr=boolean
  Switch2 : Switch  Criteria=u2 ~= 0  OutDataTypeStr=boolean
  flag : Outport  OutDataTypeStr=boolean
  wires:
  flag_old/1 -> Switch2/3
  Switch1/1 -> flag/1
  Constant1/1 -> Switch2/1
  hys/1 -> Add/2
  Add/1 -> Relational Operator1/2
  Relational Operator1/1 -> Switch2/2
  Switch2/1 -> Switch1/3
  Constant/1 -> Switch1/1
  Relational Operator3/1 -> Switch1/2
  cal/1 -> Add/1, Relational Operator3/2
  val/1 -> Relational Operator3/1, Relational Operator1/1

== system TRAMI_DCT_AT/TCU_Main/ShiftScheduleControl/ShiftScheduleControl/TCU_Shift_Schedule/Subsystem ==
  gear_shift_map_old : Inport  OutDataTypeStr=int16
  v_vehicle : Inport  Port=2  OutDataTypeStr=single
  v_shift_9A : Inport  Port=3  OutDataTypeStr=single
  v_shift_A9 : Inport  Port=4  OutDataTypeStr=single
  elseif_Input5 : Inport  Port=5  OutDataTypeStr=int16
  Constant2 : Constant  Value=10  OutDataTypeStr=int16
  Logical Operator : Logic  AllPortsSameDT=off  OutDataTypeStr=boolean
  Logical Operator1 : Logic  Operator=OR  AllPortsSameDT=off  OutDataTypeStr=boolean
  Logical Operator2 : Logic  AllPortsSameDT=off  OutDataTypeStr=boolean
  Relational Operator3 : RelationalOperator  Operator=<=  OutDataTypeStr=boolean  RndMeth=Nearest
  Relational Operator4 : RelationalOperator  OutDataTypeStr=boolean  RndMeth=Nearest
  Relational Operator5 : RelationalOperator  Operator===  OutDataTypeStr=boolean  RndMeth=Nearest
  Relational Operator6 : RelationalOperator  OutDataTypeStr=boolean  RndMeth=Nearest
  Switch1 : Switch  Criteria=u2 ~= 0  OutDataTypeStr=int16
  Out1 : Outport  OutDataTypeStr=int16
  wires:
  Logical Operator/1 -> Logical Operator1/1
  Logical Operator2/1 -> Logical Operator1/2
  Relational Operator3/1 -> Logical Operator/1
  Relational Operator5/1 -> Logical Operator2/1
  Constant2/1 -> Switch1/1, Relational Operator3/2, Relational Operator5/2
  Relational Operator4/1 -> Logical Operator/2
  Logical Operator1/1 -> Switch1/2
  Switch1/1 -> Out1/1
  elseif_Input5/1 -> Switch1/3
  Relational Operator6/1 -> Logical Operator2/2
  gear_shift_map_old/1 -> Relational Operator5/1, Relational Operator3/1
  v_vehicle/1 -> Relational Operator6/1, Relational Operator4/1
  v_shift_9A/1 -> Relational Operator4/2
  v_shift_A9/1 -> Relational Operator6/2

== system TRAMI_DCT_AT/TCU_Main/ShiftScheduleControl/ShiftScheduleControl/TCU_Shift_Schedule/Subsystem1 ==
  gear_shift_map_old : Inport  OutDataTypeStr=int16
  v_vehicle : Inport  Port=2  OutDataTypeStr=single
  v_shift_89 : Inport  Port=3  OutDataTypeStr=single
  v_shift_98 : Inport  Port=4  OutDataTypeStr=single
  elseif_Input5 : Inport  Port=5  OutDataTypeStr=int16
  Constant2 : Constant  Value=9  OutDataTypeStr=int16
  Logical Operator : Logic  AllPortsSameDT=off  OutDataTypeStr=boolean
  Logical Operator1 : Logic  Operator=OR  AllPortsSameDT=off  OutDataTypeStr=boolean
  Logical Operator2 : Logic  AllPortsSameDT=off  OutDataTypeStr=boolean
  Relational Operator3 : RelationalOperator  Operator=<=  OutDataTypeStr=boolean  RndMeth=Nearest
  Relational Operator4 : RelationalOperator  OutDataTypeStr=boolean  RndMeth=Nearest
  Relational Operator5 : RelationalOperator  OutDataTypeStr=boolean  RndMeth=Nearest
  Relational Operator6 : RelationalOperator  OutDataTypeStr=boolean  RndMeth=Nearest
  Switch1 : Switch  Criteria=u2 ~= 0  OutDataTypeStr=int16
  Out1 : Outport  OutDataTypeStr=int16
  wires:
  v_shift_98/1 -> Relational Operator6/2
  v_shift_89/1 -> Relational Operator4/2
  v_vehicle/1 -> Relational Operator4/1, Relational Operator6/1
  gear_shift_map_old/1 -> Relational Operator3/1, Relational Operator5/1
  Relational Operator6/1 -> Logical Operator2/2
  elseif_Input5/1 -> Switch1/3
  Switch1/1 -> Out1/1
  Logical Operator1/1 -> Switch1/2
  Relational Operator4/1 -> Logical Operator/2
  Relational Operator5/1 -> Logical Operator2/1
  Relational Operator3/1 -> Logical Operator/1
  Logical Operator2/1 -> Logical Operator1/2
  Logical Operator/1 -> Logical Operator1/1
  Constant2/1 -> Relational Operator5/2, Relational Operator3/2, Switch1/1

== system TRAMI_DCT_AT/TCU_Main/ShiftScheduleControl/ShiftScheduleControl/TCU_Shift_Schedule/Subsystem2 ==
  gear_shift_map_old : Inport  OutDataTypeStr=int16
  v_vehicle : Inport  Port=2  OutDataTypeStr=single
  v_shift_78 : Inport  Port=3  OutDataTypeStr=single
  v_shift_87 : Inport  Port=4  OutDataTypeStr=single
  elseif_Input5 : Inport  Port=5  OutDataTypeStr=int16
  Constant2 : Constant  Value=8  OutDataTypeStr=int16
  Logical Operator : Logic  AllPortsSameDT=off  OutDataTypeStr=boolean
  Logical Operator1 : Logic  Operator=OR  AllPortsSameDT=off  OutDataTypeStr=boolean
  Logical Operator2 : Logic  AllPortsSameDT=off  OutDataTypeStr=boolean
  Relational Operator3 : RelationalOperator  Operator=<=  OutDataTypeStr=boolean  RndMeth=Nearest
  Relational Operator4 : RelationalOperator  OutDataTypeStr=boolean  RndMeth=Nearest
  Relational Operator5 : RelationalOperator  OutDataTypeStr=boolean  RndMeth=Nearest
  Relational Operator6 : RelationalOperator  OutDataTypeStr=boolean  RndMeth=Nearest
  Switch1 : Switch  Criteria=u2 ~= 0  OutDataTypeStr=int16
  Out1 : Outport  OutDataTypeStr=int16
  wires:
  Logical Operator/1 -> Logical Operator1/1
  Logical Operator2/1 -> Logical Operator1/2
  Relational Operator3/1 -> Logical Operator/1
  Relational Operator5/1 -> Logical Operator2/1
  Relational Operator4/1 -> Logical Operator/2
  Logical Operator1/1 -> Switch1/2
  Switch1/1 -> Out1/1
  elseif_Input5/1 -> Switch1/3
  Relational Operator6/1 -> Logical Operator2/2
  gear_shift_map_old/1 -> Relational Operator5/1, Relational Operator3/1
  v_vehicle/1 -> Relational Operator6/1, Relational Operator4/1
  v_shift_78/1 -> Relational Operator4/2
  v_shift_87/1 -> Relational Operator6/2
  Constant2/1 -> Switch1/1, Relational Operator3/2, Relational Operator5/2

== system TRAMI_DCT_AT/TCU_Main/ShiftScheduleControl/ShiftScheduleControl/TCU_Shift_Schedule/Subsystem3 ==
  gear_shift_map_old1 : Inport  OutDataTypeStr=int16
  v_vehicle1 : Inport  Port=2  OutDataTypeStr=single
  v_shift_1 : Inport  Port=3  OutDataTypeStr=single
  v_shift_2 : Inport  Port=4  OutDataTypeStr=single
  elseif_Input1 : Inport  Port=5  OutDataTypeStr=int16
  Constant1 : Constant  Value=7  OutDataTypeStr=int16
  Logical Operator3 : Logic  AllPortsSameDT=off  OutDataTypeStr=boolean
  Logical Operator4 : Logic  Operator=OR  AllPortsSameDT=off  OutDataTypeStr=boolean
  Logical Operator5 : Logic  AllPortsSameDT=off  OutDataTypeStr=boolean
  Relational Operator1 : RelationalOperator  Operator=<=  OutDataTypeStr=boolean  RndMeth=Nearest
  Relational Operator2 : RelationalOperator  OutDataTypeStr=boolean  RndMeth=Nearest
  Relational Operator7 : RelationalOperator  OutDataTypeStr=boolean  RndMeth=Nearest
  Relational Operator8 : RelationalOperator  OutDataTypeStr=boolean  RndMeth=Nearest
  Switch2 : Switch  Criteria=u2 ~= 0  OutDataTypeStr=int16
  Out2 : Outport  OutDataTypeStr=int16
  wires:
  v_shift_1/1 -> Relational Operator2/2
  Relational Operator8/1 -> Logical Operator5/2
  Switch2/1 -> Out2/1
  Logical Operator4/1 -> Switch2/2
  Relational Operator2/1 -> Logical Operator3/2
  v_shift_2/1 -> Relational Operator8/2
  Constant1/1 -> Switch2/1, Relational Operator7/2, Relational Operator1/2
  Relational Operator1/1 -> Logical Operator3/1
  v_vehicle1/1 -> Relational Operator2/1, Relational Operator8/1
  gear_shift_map_old1/1 -> Relational Operator7/1, Relational Operator1/1
  Logical Operator3/1 -> Logical Operator4/1
  elseif_Input1/1 -> Switch2/3
  Logical Operator5/1 -> Logical Operator4/2
  Relational Operator7/1 -> Logical Operator5/1

== system TRAMI_DCT_AT/TCU_Main/ShiftScheduleControl/ShiftScheduleControl/TCU_Shift_Schedule/Subsystem4 ==
  gear_shift_map_old : Inport  OutDataTypeStr=int16
  v_vehicle : Inport  Port=2  OutDataTypeStr=single
  v_shift_56 : Inport  Port=3  OutDataTypeStr=single
  v_shift_65 : Inport  Port=4  OutDataTypeStr=single
  elseif_Input5 : Inport  Port=5  OutDataTypeStr=int16
  Constant2 : Constant  Value=6  OutDataTypeStr=int16
  Logical Operator : Logic  AllPortsSameDT=off  OutDataTypeStr=boolean
  Logical Operator1 : Logic  Operator=OR  AllPortsSameDT=off  OutDataTypeStr=boolean
  Logical Operator2 : Logic  AllPortsSameDT=off  OutDataTypeStr=boolean
  Relational Operator3 : RelationalOperator  Operator=<=  OutDataTypeStr=boolean  RndMeth=Nearest
  Relational Operator4 : RelationalOperator  OutDataTypeStr=boolean  RndMeth=Nearest
  Relational Operator5 : RelationalOperator  OutDataTypeStr=boolean  RndMeth=Nearest
  Relational Operator6 : RelationalOperator  OutDataTypeStr=boolean  RndMeth=Nearest
  Switch1 : Switch  Criteria=u2 ~= 0  OutDataTypeStr=int16
  Out1 : Outport  OutDataTypeStr=int16
  wires:
  Logical Operator/1 -> Logical Operator1/1
  Logical Operator2/1 -> Logical Operator1/2
  Relational Operator3/1 -> Logical Operator/1
  Relational Operator5/1 -> Logical Operator2/1
  Constant2/1 -> Relational Operator5/2, Relational Operator3/2, Switch1/1
  Relational Operator4/1 -> Logical Operator/2
  Logical Operator1/1 -> Switch1/2
  Switch1/1 -> Out1/1
  elseif_Input5/1 -> Switch1/3
  Relational Operator6/1 -> Logical Operator2/2
  gear_shift_map_old/1 -> Relational Operator3/1, Relational Operator5/1
  v_vehicle/1 -> Relational Operator6/1, Relational Operator4/1
  v_shift_56/1 -> Relational Operator4/2
  v_shift_65/1 -> Relational Operator6/2

== system TRAMI_DCT_AT/TCU_Main/ShiftScheduleControl/ShiftScheduleControl/TCU_Shift_Schedule/Subsystem5 ==
  gear_shift_map_old : Inport  OutDataTypeStr=int16
  v_vehicle : Inport  Port=2  OutDataTypeStr=single
  v_shift_45 : Inport  Port=3  OutDataTypeStr=single
  v_shift_54 : Inport  Port=4  OutDataTypeStr=single
  elseif_Input5 : Inport  Port=5  OutDataTypeStr=int16
  Constant2 : Constant  Value=5  OutDataTypeStr=int16
  Logical Operator : Logic  AllPortsSameDT=off  OutDataTypeStr=boolean
  Logical Operator1 : Logic  Operator=OR  AllPortsSameDT=off  OutDataTypeStr=boolean
  Logical Operator2 : Logic  AllPortsSameDT=off  OutDataTypeStr=boolean
  Relational Operator3 : RelationalOperator  Operator=<=  OutDataTypeStr=boolean  RndMeth=Nearest
  Relational Operator4 : RelationalOperator  OutDataTypeStr=boolean  RndMeth=Nearest
  Relational Operator5 : RelationalOperator  OutDataTypeStr=boolean  RndMeth=Nearest
  Relational Operator6 : RelationalOperator  OutDataTypeStr=boolean  RndMeth=Nearest
  Switch1 : Switch  Criteria=u2 ~= 0  OutDataTypeStr=int16
  Out1 : Outport  OutDataTypeStr=int16
  wires:
  v_shift_54/1 -> Relational Operator6/2
  v_shift_45/1 -> Relational Operator4/2
  v_vehicle/1 -> Relational Operator4/1, Relational Operator6/1
  gear_shift_map_old/1 -> Relational Operator3/1, Relational Operator5/1
  Relational Operator6/1 -> Logical Operator2/2
  elseif_Input5/1 -> Switch1/3
  Switch1/1 -> Out1/1
  Logical Operator1/1 -> Switch1/2
  Relational Operator4/1 -> Logical Operator/2
  Constant2/1 -> Relational Operator3/2, Relational Operator5/2, Switch1/1
  Relational Operator5/1 -> Logical Operator2/1
  Relational Operator3/1 -> Logical Operator/1
  Logical Operator2/1 -> Logical Operator1/2
  Logical Operator/1 -> Logical Operator1/1

== system TRAMI_DCT_AT/TCU_Main/ShiftScheduleControl/ShiftScheduleControl/TCU_Shift_Schedule/Subsystem6 ==
  gear_shift_map_old : Inport  OutDataTypeStr=int16
  v_vehicle : Inport  Port=2  OutDataTypeStr=single
  v_shift_34 : Inport  Port=3  OutDataTypeStr=single
  v_shift_43 : Inport  Port=4  OutDataTypeStr=single
  elseif_Input5 : Inport  Port=5  OutDataTypeStr=int16
  Constant2 : Constant  Value=4  OutDataTypeStr=int16
  Logical Operator : Logic  AllPortsSameDT=off  OutDataTypeStr=boolean
  Logical Operator1 : Logic  Operator=OR  AllPortsSameDT=off  OutDataTypeStr=boolean
  Logical Operator2 : Logic  AllPortsSameDT=off  OutDataTypeStr=boolean
  Relational Operator3 : RelationalOperator  Operator=<=  OutDataTypeStr=boolean  RndMeth=Nearest
  Relational Operator4 : RelationalOperator  OutDataTypeStr=boolean  RndMeth=Nearest
  Relational Operator5 : RelationalOperator  OutDataTypeStr=boolean  RndMeth=Nearest
  Relational Operator6 : RelationalOperator  OutDataTypeStr=boolean  RndMeth=Nearest
  Switch1 : Switch  Criteria=u2 ~= 0  OutDataTypeStr=int16
  Out1 : Outport  OutDataTypeStr=int16
  wires:
  Logical Operator/1 -> Logical Operator1/1
  Logical Operator2/1 -> Logical Operator1/2
  Relational Operator3/1 -> Logical Operator/1
  Relational Operator5/1 -> Logical Operator2/1
  Constant2/1 -> Switch1/1, Relational Operator3/2, Relational Operator5/2
  Relational Operator4/1 -> Logical Operator/2
  Logical Operator1/1 -> Switch1/2
  Switch1/1 -> Out1/1
  elseif_Input5/1 -> Switch1/3
  Relational Operator6/1 -> Logical Operator2/2
  gear_shift_map_old/1 -> Relational Operator3/1, Relational Operator5/1
  v_vehicle/1 -> Relational Operator6/1, Relational Operator4/1
  v_shift_34/1 -> Relational Operator4/2
  v_shift_43/1 -> Relational Operator6/2

== system TRAMI_DCT_AT/TCU_Main/ShiftScheduleControl/ShiftScheduleControl/TCU_Shift_Schedule/Subsystem7 ==
  gear_shift_map_old : Inport  OutDataTypeStr=int16
  v_vehicle : Inport  Port=2  OutDataTypeStr=single
  v_shift_23 : Inport  Port=3  OutDataTypeStr=single
  v_shift_32 : Inport  Port=4  OutDataTypeStr=single
  elseif_Input5 : Inport  Port=5  OutDataTypeStr=int16
  Constant2 : Constant  Value=3  OutDataTypeStr=int16
  Logical Operator : Logic  AllPortsSameDT=off  OutDataTypeStr=boolean
  Logical Operator1 : Logic  Operator=OR  AllPortsSameDT=off  OutDataTypeStr=boolean
  Logical Operator2 : Logic  AllPortsSameDT=off  OutDataTypeStr=boolean
  Relational Operator3 : RelationalOperator  Operator=<=  OutDataTypeStr=boolean  RndMeth=Nearest
  Relational Operator4 : RelationalOperator  OutDataTypeStr=boolean  RndMeth=Nearest
  Relational Operator5 : RelationalOperator  OutDataTypeStr=boolean  RndMeth=Nearest
  Relational Operator6 : RelationalOperator  OutDataTypeStr=boolean  RndMeth=Nearest
  Switch1 : Switch  Criteria=u2 ~= 0  OutDataTypeStr=int16
  Out1 : Outport  OutDataTypeStr=int16
  wires:
  v_shift_32/1 -> Relational Operator6/2
  v_shift_23/1 -> Relational Operator4/2
  v_vehicle/1 -> Relational Operator4/1, Relational Operator6/1
  gear_shift_map_old/1 -> Relational Operator3/1, Relational Operator5/1
  Relational Operator6/1 -> Logical Operator2/2
  elseif_Input5/1 -> Switch1/3
  Switch1/1 -> Out1/1
  Logical Operator1/1 -> Switch1/2
  Relational Operator4/1 -> Logical Operator/2
  Constant2/1 -> Relational Operator5/2, Relational Operator3/2, Switch1/1
  Relational Operator5/1 -> Logical Operator2/1
  Relational Operator3/1 -> Logical Operator/1
  Logical Operator2/1 -> Logical Operator1/2
  Logical Operator/1 -> Logical Operator1/1

== system TRAMI_DCT_AT/TCU_Main/ShiftScheduleControl/ShiftScheduleControl/TCU_Shift_Schedule/Subsystem8 ==
  gear_shift_map_old : Inport  OutDataTypeStr=int16
  v_vehicle : Inport  Port=2  OutDataTypeStr=single
  v_shift_12 : Inport  Port=3  OutDataTypeStr=single
  v_shift_21 : Inport  Port=4  OutDataTypeStr=single
  elseif_Input5 : Inport  Port=5  OutDataTypeStr=int16
  Constant2 : Constant  Value=2  OutDataTypeStr=int16
  Logical Operator : Logic  AllPortsSameDT=off  OutDataTypeStr=boolean
  Logical Operator1 : Logic  Operator=OR  AllPortsSameDT=off  OutDataTypeStr=boolean
  Logical Operator2 : Logic  AllPortsSameDT=off  OutDataTypeStr=boolean
  Relational Operator3 : RelationalOperator  Operator=<=  OutDataTypeStr=boolean  RndMeth=Nearest
  Relational Operator4 : RelationalOperator  OutDataTypeStr=boolean  RndMeth=Nearest
  Relational Operator5 : RelationalOperator  OutDataTypeStr=boolean  RndMeth=Nearest
  Relational Operator6 : RelationalOperator  OutDataTypeStr=boolean  RndMeth=Nearest
  Switch1 : Switch  Criteria=u2 ~= 0  OutDataTypeStr=int16
  Out1 : Outport  OutDataTypeStr=int16
  wires:
  Logical Operator/1 -> Logical Operator1/1
  Logical Operator2/1 -> Logical Operator1/2
  Relational Operator3/1 -> Logical Operator/1
  Relational Operator5/1 -> Logical Operator2/1
  Constant2/1 -> Relational Operator5/2, Relational Operator3/2, Switch1/1
  Relational Operator4/1 -> Logical Operator/2
  Logical Operator1/1 -> Switch1/2
  Switch1/1 -> Out1/1
  elseif_Input5/1 -> Switch1/3
  Relational Operator6/1 -> Logical Operator2/2
  gear_shift_map_old/1 -> Relational Operator3/1, Relational Operator5/1
  v_vehicle/1 -> Relational Operator6/1, Relational Operator4/1
  v_shift_12/1 -> Relational Operator4/2
  v_shift_21/1 -> Relational Operator6/2

== system TRAMI_DCT_AT/TCU_Main/StartingDeviceControl/StartingDeviceControl/TCU_Slip_Control/Table_search_3D_G1 ==
  X : Inport  OutDataTypeStr=single
  Y : Inport  Port=2  OutDataTypeStr=single
  1-D Lookup Table1 : Lookup_n-D  NumberOfTableDimensions=1  BreakpointsForDimension1=axis_x  Table=tbl_x  ExtrapMethod=Clip  InternalRulePriority=Speed  OutDataTypeStr=single  RndMeth=Simplest  InputSameDT=on
  1-D Lookup Table2 : Lookup_n-D  NumberOfTableDimensions=1  BreakpointsForDimension1=axis_y  Table=tbl_y  ExtrapMethod=Clip  InternalRulePriority=Speed  OutDataTypeStr=single  RndMeth=Simplest  InputSameDT=on
  2-D Lookup Table : Lookup_n-D  BreakpointsForDimension1=tbl_y  BreakpointsForDimension2=tbl_x  Table=map  ExtrapMethod=Clip  InternalRulePriority=Speed  OutDataTypeStr=single  RndMeth=Simplest  InputSameDT=on
  out : Outport  OutDataTypeStr=single
  wires:
  2-D Lookup Table/1 -> out/1
  X/1 -> 1-D Lookup Table1/1  "data_x"
  Y/1 -> 1-D Lookup Table2/1  "data_y"
  1-D Lookup Table2/1 -> 2-D Lookup Table/1  "y_nrm"
  1-D Lookup Table1/1 -> 2-D Lookup Table/2  "x_nrm"
